simulink model "DE_LBS_mass_2"  (R2018a)
settings: Solver=ode23t  StartTime=0.0  StopTime=50  EnableMultiTasking=on
InitFcn:
  | Parameter;
values from neighbouring files (symbols this model uses):
  task_params = struct    [run.m]
undefined symbols (not defined in the file or in its folder): A, Bd, C, Dd, initConds, params_BIAS, yeq
settings Model: Creator=Johannes  LastModifiedBy=tim
settings DataIOCC: LimitDataPoints=on  SaveFormat=Array  SignalLoggingSaveFormat=ModelDataLogs
settings OptimizationCC: LifeSpan=inf
settings DebuggingCC: UnderspecifiedInitializationDetection=Classic  MergeDetectMultiDrivingBlocksExec=none  SolverPrmCheckMsg=warning  MultiTaskDSMMsg=warning  MultiTaskCondExecSysMsg=none  SFUnexpectedBacktrackingDiag=warning  SFNoUnconditionalDefaultTransitionDiag=warning  SFExecutionAtInitializationDiag=none
settings HardwareCC: ProdBitPerPointer=32  ProdBitPerSizeT=32  ProdBitPerPtrDiffT=32  ProdLargestAtomicFloat=None  ProdIntDivRoundTo=Undefined  ProdEndianess=Unspecified  ProdWordSize=32  ProdHWDeviceType=32-bit Generic
settings ModelReferenceCC: PropagateSignalLabelsOutOfModel=off
settings CodeAppCC: StateflowObjectComments=on
settings GRTTargetCC: TargetLangStandard=C89/C90 (ANSI)  GeneratePreprocessorConditionals=Disable all
settings ConfigComp: CovMetricSettings=dw  CovHtmlReporting=on  CovSaveCumulativeToWorkspaceVar=on  CovSaveSingleToWorkspaceVar=on  CovExternalEMLEnable=off

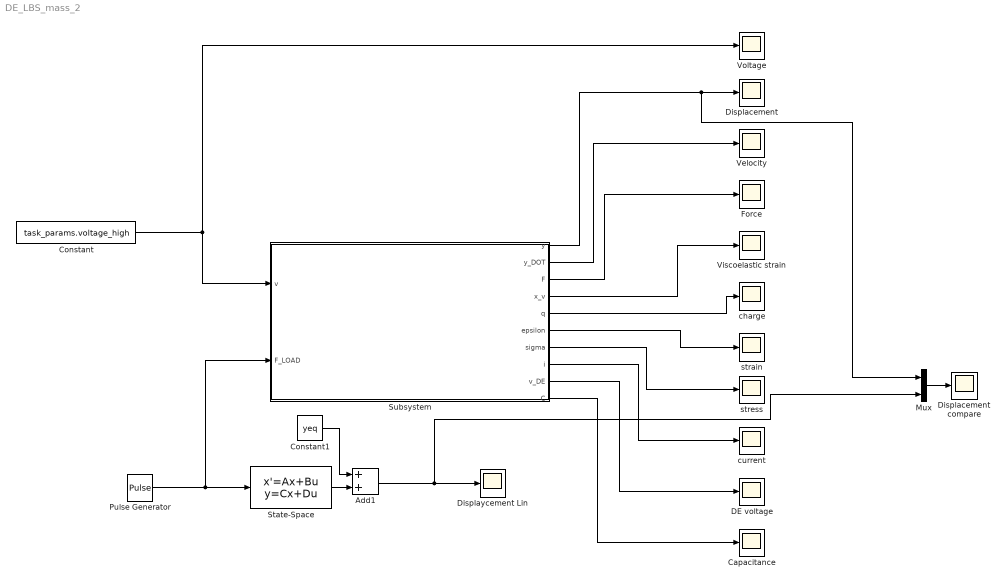
== system DE_LBS_mass_2 ==
  Add1 : Sum
  Capacitance : Scope
  Constant : Constant  Value=task_params.voltage_high
  Constant1 : Constant  Value=yeq
  DE voltage : Scope
  Displacement : Scope
  "Displacement compare " : Scope
  "Displaycement Lin " : Scope
  Force : Scope
  Mux : Mux  Inputs=2
  Pulse Generator : DiscretePulseGenerator  PulseType=Time based  Amplitude=task_params.fore  Period=5  PulseWidth=50
  State-Space : StateSpace  A=A  B=Bd  C=C  D=Dd  InitialCondition=0
  Subsystem : Subsystem
      mask Display:
      | color('black');
      | patch(4*[-1 1 1 -1],1.75*[-1 -1 1 1],[1 1 1]);
      | patch(2*[-1 1 1 -1],1.2*[-1 -1 1 1],[0 0 0]);
      | patch(1.95*[-1 1 1 -1],0.8*[-1 -1 1 1],[1 1 1]);
      | disp('DE LBS mass');
      | 
      | color('blue');
      | port_label('input', 1, 'v [V]','texmode','on');
      | port_label('input', 2, 'F_{LOAD} [N]','texmode','on');
      | 
      | color('red');
      | port_label('output', 1, 'y [m]','texmode','on');
      | port_label('output', 2, 'y_{dot} [m/s]','texmode','on');
      | port_label('output', 3, 'F [N]','texmode','on');
      | port_label('output', 4, 'x_v [-]','texmode','on');
      | port_label('output', 5, 'q [C]','texmode','on');
      | port_label('output', 6, '\epsilon_1 [-]','texmode','on');
      | port_label('output', 7, '\sigma_1 [Pa]','texmode','on');
      | port_label('output', 8, 'i [A]','texmode','on');
      | port_label('output', 9, 'v_{DE} [V]','texmode','on');
      | port_label('output', 10, 'C [F]','texmode','on');
  Velocity : Scope
  Viscoelastic strain : Scope
  Voltage : Scope
  charge : Scope
  current : Scope
  strain : Scope
  stress : Scope
  wires:
  Pulse Generator/1 -> Subsystem/2(F_LOAD), State-Space/1
  Subsystem/3(F) -> Force/1
  Subsystem/4(x_v) -> Viscoelastic strain/1
  Subsystem/5(q) -> charge/1
  Subsystem/6(epsilon) -> strain/1
  Subsystem/7(sigma) -> stress/1
  Subsystem/8(i) -> current/1
  Subsystem/9(v_DE) -> DE voltage/1
  Subsystem/10(C) -> Capacitance/1
  Subsystem/1(y) -> Mux/1, Displacement/1
  Subsystem/2(y_DOT) -> Velocity/1
  Constant/1 -> Voltage/1, Subsystem/1(v)
  Mux/1 -> "Displacement compare "/1
  Constant1/1 -> Add1/1
  State-Space/1 -> Add1/2
  Add1/1 -> Mux/2, "Displaycement Lin "/1

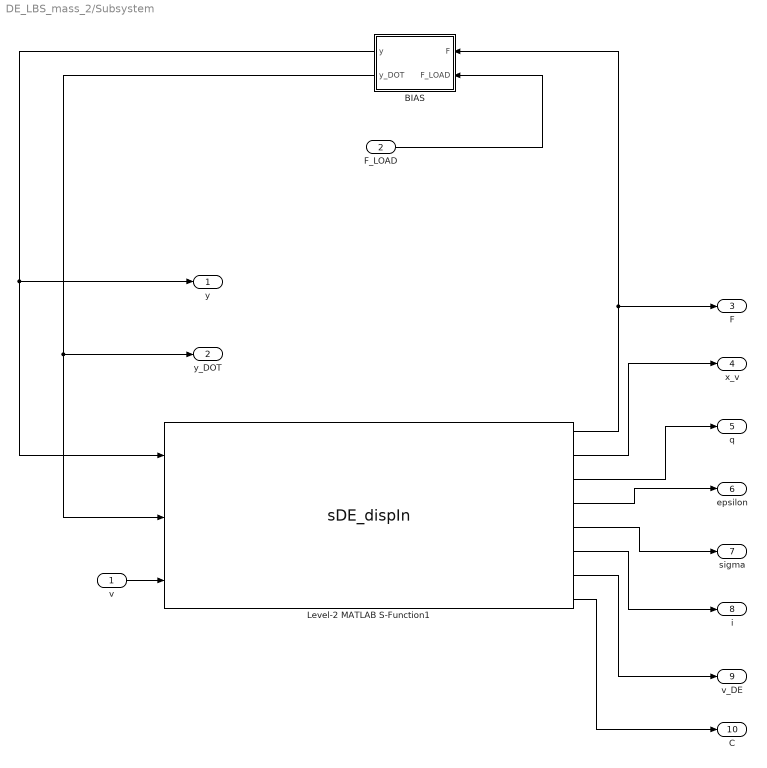
== system DE_LBS_mass_2/Subsystem ==
  v : Inport
  F_LOAD : Inport  Port=2
  BIAS : Subsystem
  Level-2 MATLAB S-Function1 : M-S-Function  FunctionName=sDE_dispIn  Parameters=params, initConds
      mask Display:
      | color('black');
      | patch(4*[-1 1 1 -1],1.75*[-1 -1 1 1],[1 1 1]);
      | patch(2*[-1 1 1 -1],1.2*[-1 -1 1 1],[0 0 0]);
      | patch(1.95*[-1 1 1 -1],0.8*[-1 -1 1 1],[1 1 1]);
      | disp('DE');
      | 
      | color('blue');
      | port_label('input', 1, 'y [m]','texmode','on');
      | port_label('input', 2, 'y_{dot} [m/s]','texmode','on');
      | port_label('input', 3, 'v [V]','texmode','on');
      | 
      | color('red');
      | port_label('output', 1, 'F [N]','texmode','on');
      | port_label('output', 2, 'x_v [-]','texmode','on');
      | port_label('output', 3, 'q [C]','texmode','on');
      | port_label('output', 4, '\epsilon_1 [-]','texmode','on');
      | port_label('output', 5, '\sigma_1 [Pa]','texmode','on');
      | port_label('output', 6, 'i [A]','texmode','on');
      | port_label('output', 7, 'v_{DE} [V]','texmode','on');
      | port_label('output', 8, 'C [F]','texmode','on');
  y : Outport
  y_DOT : Outport  Port=2
  F : Outport  Port=3
  x_v : Outport  Port=4
  q : Outport  Port=5
  epsilon : Outport  Port=6
  sigma : Outport  Port=7
  i : Outport  Port=8
  v_DE : Outport  Port=9
  C : Outport  Port=10
  wires:
  v/1 -> Level-2 MATLAB S-Function1/3
  Level-2 MATLAB S-Function1/7 -> v_DE/1
  Level-2 MATLAB S-Function1/1 -> BIAS/1(F), F/1
  Level-2 MATLAB S-Function1/3 -> q/1
  Level-2 MATLAB S-Function1/4 -> epsilon/1
  Level-2 MATLAB S-Function1/5 -> sigma/1
  Level-2 MATLAB S-Function1/8 -> C/1
  Level-2 MATLAB S-Function1/6 -> i/1
  Level-2 MATLAB S-Function1/2 -> x_v/1
  BIAS/1(y) -> y/1, Level-2 MATLAB S-Function1/1
  BIAS/2(y_DOT) -> y_DOT/1, Level-2 MATLAB S-Function1/2
  F_LOAD/1 -> BIAS/2(F_LOAD)

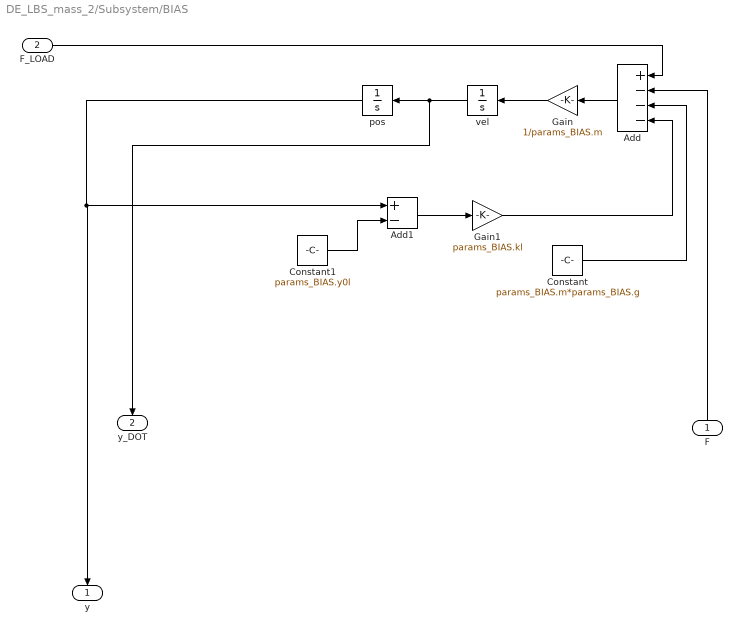
== system DE_LBS_mass_2/Subsystem/BIAS ==
  F : Inport
  F_LOAD : Inport  Port=2
  Add : Sum  Inputs=+---
  Add1 : Sum  Inputs=+-
  Constant : Constant  Value=params_BIAS.m*params_BIAS.g
  Constant1 : Constant  Value=params_BIAS.y0l
  Gain : Gain  Gain=1/params_BIAS.m
  Gain1 : Gain  Gain=params_BIAS.kl
  pos : Integrator  InitialCondition=initConds.y
  vel : Integrator  InitialCondition=initConds.y_dot
  y : Outport
  y_DOT : Outport  Port=2
  wires:
  F_LOAD/1 -> Add/1
  vel/1 -> y_DOT/1, pos/1
  Gain/1 -> vel/1
  pos/1 -> y/1, Add1/1
  Gain1/1 -> Add/4
  Add/1 -> Gain/1
  Constant/1 -> Add/3
  Add1/1 -> Gain1/1
  Constant1/1 -> Add1/2
  F/1 -> Add/2
